simulink model "mSingleTorsionalCompliance"  (R2019b)
settings: Solver=ode23tb  StartTime=0.0  StopTime=10  FixedStep=.001  RelTol=1e-3
libraries: VsrLibCoupling x1
settings Model: Creator=9bt  LastModifiedBy=4qz

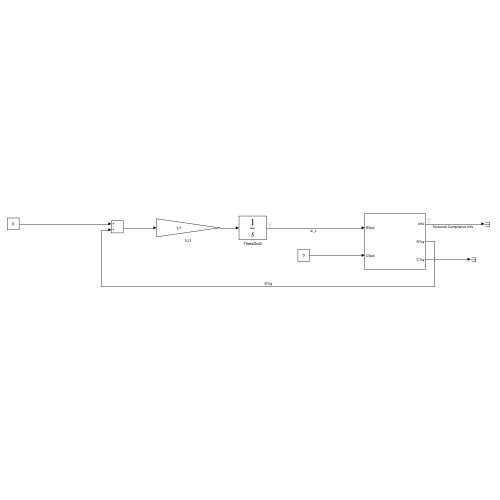
[thumbnail: Simulink's stored preview of the top-level diagram]
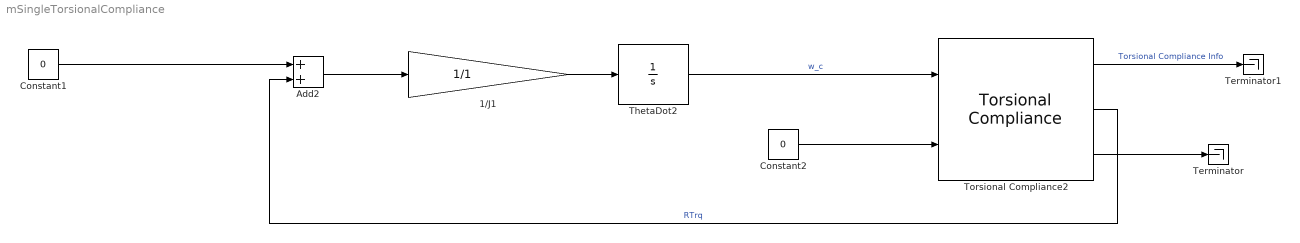
== system mSingleTorsionalCompliance ==
  1/J1 : Gain  Gain=1/1
  Add2 : Sum
  Constant1 : Constant  Value=0
  Constant2 : Constant  Value=0
  Terminator : Terminator
  Terminator1 : Terminator
  ThetaDot2 : Integrator  InitialCondition=1
  Torsional Compliance2 : VsrLibCoupling/Torsional Compliance  StiffnessCalcMethodPopup=Shaft dimensions and material properties  DampingCalcMethodPopup=Damping ratio  D_o=.02  D_i=.015  L_shaft=.5  G=77e9  Jcalc=1  zeta=2  wn=40.6649  wd=0  k=1653.6313  b=1000  omega_c=500  theta_0=0  omega_0=0
  wires:
  ThetaDot2/1 -> Torsional Compliance2/1  "w_c"
  Add2/1 -> 1/J1/1
  Constant1/1 -> Add2/1
  1/J1/1 -> ThetaDot2/1
  Torsional Compliance2/2 -> Add2/2  "RTrq"
  Constant2/1 -> Torsional Compliance2/2
  Torsional Compliance2/3 -> Terminator/1
  Torsional Compliance2/1 -> Terminator1/1  "Torsional Compliance Info"
